simulink model "EuroNCAP_AEB_VRU_reversing_adult_stationary_cs"  (R2014b)
settings: Solver=ode5  SolverMode=SingleTasking  StartTime=0.0  StopTime=100  FixedStep=1/100  RelTol=1e-3
PreLoadFcn:
  | mbxruntime.callbacks.PreLoadFcn(bdroot);
  | check_NUTS_defined;
  | 
  | assignin('base',['model_closed_' bdroot],false);
  | 
  | addpath('../includes_PPS');
PostLoadFcn:
  | mbxruntime.callbacks.PostLoadFcn(bdroot);
InitFcn:
  | mbxruntime.callbacks.InitFcn(bdroot);
  | 
  | % Define simulink variables if they
  | % do not exist
  | if ~exist('HostVelocity', 'var')
  |   HostVelocity = 4;
  | end
  | 
  | if ~exist('Offset', 'var')
  |  Offset = 0;
  | end
StartFcn:
  | mbxruntime.callbacks.StartFcn(bdroot);
StopFcn:
  | mbxruntime.callbacks.StopFcn(bdroot);
model workspace: external: MAT-File .\EuroNCAP_AEB_VRU_reversing_adult_stationary_cs_hws.mat (data not in the file)
undefined symbols (not defined in the file or in its folder): mbxruntime, tabledata, warningInitialVelocity, x0
undefined symbols (not defined in the file): EuroNCAP_AEB_VRU_reversing_adult_stationary_cs_1d213d8ad9f41b81, EuroNCAP_AEB_VRU_reversing_adult_stationary_cs_23249e0323da09f5, EuroNCAP_AEB_VRU_reversing_adult_stationary_cs_24cc001f49944e92, EuroNCAP_AEB_VRU_reversing_adult_stationary_cs_285ecd3c3433122b, EuroNCAP_AEB_VRU_reversing_adult_stationary_cs_592b93520602ee78, EuroNCAP_AEB_VRU_reversing_adult_stationary_cs_7caeaf879e7765e9, EuroNCAP_AEB_VRU_reversing_adult_stationary_cs_93da770b460b611e, EuroNCAP_AEB_VRU_reversing_adult_stationary_cs_a0ea79e870de98f7, EuroNCAP_AEB_VRU_reversing_adult_stationary_cs_abfe9a01e22132d5, EuroNCAP_AEB_VRU_reversing_adult_stationary_cs_c7aa8805d7c8ab2f, EuroNCAP_AEB_VRU_reversing_adult_stationary_cs_c9a05fd8fd346e46, EuroNCAP_AEB_VRU_reversing_adult_stationary_cs_d44be614cd41bc1c, EuroNCAP_AEB_VRU_reversing_adult_stationary_cs_d8757d69723733e9, WheelL0, WheelL1, WheelR0, WheelR1
libraries: simulink x23, PreScanUsefulBlocks x19, simulink_extras x7, PreScanSimulinkLibrary x6
(part 1 of 5)
CloseFcn:
  | mbxruntime.callbacks.CloseFcn(bdroot);
  | evalin('base',['clear model_closed_' bdroot]);
settings Model: Creator=PRESCAN  LastModifiedBy=jenkins
settings DataIOCC: SignalLoggingSaveFormat=ModelDataLogs
settings OptimizationCC: InlineParams=on  ExpressionDepthLimit=2147483647  InitFltsAndDblsToZero=on
settings DebuggingCC: SaveWithParameterizedLinksMsg=none  UnderspecifiedInitializationDetection=Classic  MergeDetectMultiDrivingBlocksExec=none  SignalResolutionControl=TryResolveAllWithWarning  SolverPrmCheckMsg=none  MultiTaskDSMMsg=warning  MultiTaskCondExecSysMsg=none  FcnCallInpInsideContextMsg=UseLocalSettings  StateNameClashWarn=warning
settings ModelReferenceCC: UpdateModelReferenceTargets=IfOutOfDate
settings SFSimCC: SimParseCustomCode=off
settings SFSimCC: SimCustomHeaderCode=|
  | #include "prescan.h"
  | #include "prescan_platform.h"
settings RTWCC: IncludeERTFirstTime=on
settings GRTTargetCC: TargetFcnLib=ansi_tfl_tmw.mat  CombineOutputUpdateFcns=off  GRTInterface=on

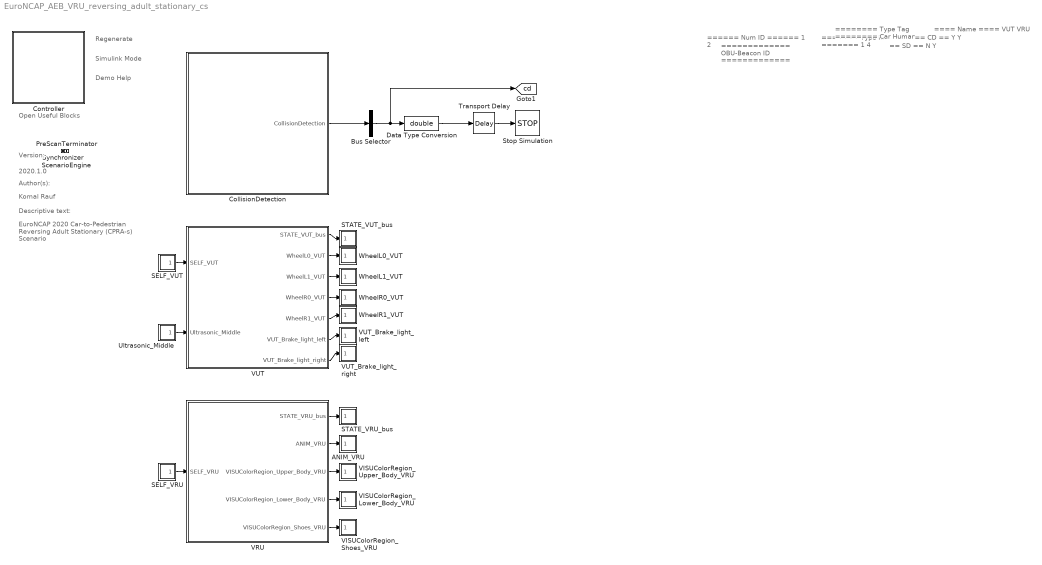
== system EuroNCAP_AEB_VRU_reversing_adult_stationary_cs ==
  note: Regenerate
  note: Simulink Mode
  note: Open Useful Blocks
  note: 2020.1.0
  note: Version:
  note: Author(s):
  note: Komal Rauf
  note: Descriptive text:
  note: EuroNCAP 2020 Car-to-Pedestrian
      | Reversing Adult Stationary
      | (CPRA-s) Scenario
  note: Demo Help
  note: ======
      | Num ID
      | ======
      | 1
      | 2
  note: =============
      | OBU-Beacon ID
      | =============
  note: =======
      | Type ID
      | =======
      | 1
      | 4
  note: ========
      | Type Tag
      | ========
      | Car
      | Human
  note: ==
      | SD
      | ==
      | N
      | Y
  note: ==
      | CD
      | ==
      | Y
      | Y
  note: ====
      | Name
      | ====
      | VUT
      | VRU
  ANIM_VRU : Subsystem  Tag=actuator/AnimationOutport  Priority=0  LoadFcn=load('PreScanAnimActuatorData.mat')  mask(PreScan Sink Block: State Animation){}
      mask help: The Human Animation port allows the human to walk, run or bend
      settings: OpenFcn=open_system([gcb '/Actuator'],'mask')
      mask Help: eval('openHelp(239)')
      mask Display: image(imread('HumanAnimated.jpg'))
  Bus Selector : BusSelector  OutputSignals=HEADER.valid
  CollisionDetection : Subsystem  Tag=sensor/CollisionDetection  Priority=30  LoadFcn=load('PrescanCollisionDetectionData.mat');load('PrescanCollisionDetectionMessage.mat')  mask(PreScan Source Block: CollisionDetection){}
      mask help: Collision Detection can be used to detect collisions between PreScan components. For Collision Detection the actual component shape is taken into account, so it is not a bounding box approach.
      settings: OpenFcn=open_system([gcb '/Sensor'],'mask')
      mask Help: eval('openHelp(811)')
      mask Display: image(imread('crash.jpg'))
  Controller : Subsystem  Description=8A3CD2955739A82C886C20AE3E253D78460D53180EE2C1B14CC08DF75A70BE77  Priority=-1  LoadFcn=load PreScanControllerData  mask(PreScan Simulation Controller){prescanversion='2020.1.0', ModelReferencing=off, TimeStep=1/100, ControlMode=0, PreScanExecutionMode=on, ControllerCount=0, ControllerIndex=0, ControllerOptions=''}
      mask prompts: prescanversion "PreScan Version"; ModelReferencing "Use Model Referencing"; TimeStep "Upload Period [s]"; ControlMode "Control Mode"; PreScanExecutionMode "Execution Mode"; ControllerCount "Controller Count"; ControllerIndex "Controller Index"; ControllerOptions "Controller Options"
      mask help:
      | Please do not remove this block from the compilation sheet,
      | as it connects the model to the PreScan environment.
      mask init:
      | model = bdroot(gcb);
      | ExperimentFile = mbxruntime.findExperimentFile(model,true); %relative path
      | 
      | [d1, d2, d3, prescandata] = prescan_Settings();
      | ModelDepo = fullfile(prescandata,'ModelDepo'); 
      | 
      | RTmode = mbxruntime.getRTMode(model);
      | 
      | SimulationMode = get_param(bdroot,'SimulationMode');
      | if strcmp(SimulationMode, 'rapid-accelerator')
      |     SimulationMode = 'external';
      | end
      | TargetName = get_param(bdroot,'SystemTargetFile');
      settings: ModelCloseFcn=assignin('base',['model_closed_' bdroot],true);
      mask Help: eval('openHelp(812)')
      mask Display: image(imread('prescanlogo.ico'))
  Data Type Conversion : DataTypeConversion  OutDataTypeStr=double
  PreScanTerminator : Subsystem  Tag=PreScanTerminator  Priority=999  LoadFcn=load PrescanTerminatorData  mask(PreScan Simulation Terminator){TimeStep=1/100}
      mask prompts: TimeStep "Upload Period [s]"
      mask help:
      | Please do not remove this block from the compilation sheet as it
      | connects the model to the PreScan environment.
      mask Help: eval('openHelp(812)')
      mask Display: image(imread('prescanlogo.ico'))
  SELF_VRU : Subsystem  Tag=sensor/SelfPort  Priority=30  LoadFcn=load('PreScanSelfSensorData.mat')  mask(PreScan Source Block: SELF){}
      mask help:
      | The SELF port shows (state) information of the actor itself. The outputs are position in the experiment's axis system and the GPS coordinates, and the object's absolute velocity and compass heading.
      |
      | For more information, please click Help.
      settings: OpenFcn=open_system([gcb '/Sensor'],'mask')
      mask Help: eval('openHelp(462)')
      mask Display: image(imread('GPS.png'))
  SELF_VUT : Subsystem  Tag=sensor/SelfPort  Priority=30  LoadFcn=load('PreScanSelfSensorData.mat')  mask(PreScan Source Block: SELF){}
      mask help:
      | The SELF port shows (state) information of the actor itself. The outputs are position in the experiment's axis system and the GPS coordinates, and the object's absolute velocity and compass heading.
      |
      | For more information, please click Help.
      settings: OpenFcn=open_system([gcb '/Sensor'],'mask')
      mask Help: eval('openHelp(462)')
      mask Display: image(imread('GPS.png'))
  STATE_VRU_bus : Subsystem  Tag=actuator/StatePort  Priority=0  LoadFcn=load('PreScanStateActuatorData.mat')  mask(PreScan Sink Block: State){}
      mask help:
      | The Actor State contains a vector signal of size (9x1), containing the following signals:
      |
      | -  Position    	(x,y,z)             	[m]
      | -  Velocity    	(vx,vy,vz)         	[m/s]
      | -  Angles       	(Roll, Pitch, Yaw)	[rad]
      |
      | The Actor state is defined in the global axis system.
      | The state is superponed on the Initial position defined in the GUI.
      |
      | For more information, please click Help.
      settings: OpenFcn=open_system([gcb '/Actuator'],'mask')
      mask Help: eval('openHelp(222)')
      mask Display: image(imread('State.png'))
  STATE_VUT_bus : Subsystem  Tag=actuator/StatePort  Priority=0  LoadFcn=load('PreScanStateActuatorData.mat')  mask(PreScan Sink Block: State){}
      mask help:
      | The Actor State contains a vector signal of size (9x1), containing the following signals:
      |
      | -  Position    	(x,y,z)             	[m]
      | -  Velocity    	(vx,vy,vz)         	[m/s]
      | -  Angles       	(Roll, Pitch, Yaw)	[rad]
      |
      | The Actor state is defined in the global axis system.
      | The state is superponed on the Initial position defined in the GUI.
      |
      | For more information, please click Help.
      settings: OpenFcn=open_system([gcb '/Actuator'],'mask')
      mask Help: eval('openHelp(222)')
      mask Display: image(imread('State.png'))
  ScenarioEngine : Subsystem  Tag=PreScanOpenScenarioBlock  Priority=10  LoadFcn=load PrescanSynchronizeData  mask(PreScan Simulation Core Block){TimeStep=1/100}
      mask prompts: TimeStep "Timestep [s]"
      mask help:
      | Please do not remove this block from the PreScan compilation sheet,
      | as it contains essential configuration parameters for a PreScan simulation.
      settings: DeleteFcn=PreScanBlockDeleteFcn;
      mask Display: image(imread('prescanlogo.ico'))
  Stop Simulation : Stop
  Synchronizer : Subsystem  Tag=PreScanSynchronizer  Priority=20  LoadFcn=load PrescanSynchronizeData  mask(PreScan Simulation Core Block){TimeStep=1/100}
      mask prompts: TimeStep "Timestep [s]"
      mask help:
      | Please do not remove this block from the PreScan compilation sheet,
      | as it contains essential configuration parameters for a PreScan simulation.
      settings: DeleteFcn=PreScanBlockDeleteFcn;
      mask Display: image(imread('prescanlogo.ico'))
  Transport Delay : TransportDelay  DelayTime=1/100
  Ultrasonic_Middle : Subsystem  Tag=sensor/UltraSonic  Priority=30  LoadFcn=load('PrescanScannerSensorData.mat');load('PrescanScannerSensorMessage.mat')  mask(PreScan Source Block: UltraSonic Sensor){}
      mask help:
      | The UltraSonic Sensor is a scanner device used to detect obstacles like cars, motor cycles, and pedestrians.
      |
      | For more information, please click Help.
      settings: OpenFcn=open_system([gcb '/Sensor'],'mask')
      mask Help: eval('openHelp(1465)')
      mask Display: image(imread('UltraSonic.png'))
  VISUColorRegion_Lower_Body_VRU : Subsystem  Tag=actuator/ColorRegion  Priority=0  LoadFcn=load('PrescanColorData')  mask(PreScan Sink Block: VisuTextureColor){}
      mask help:
      | The VisuTextureColor block provides a way to adapt the color of a vehicle.
      |
      | For more information, please click Help.
      settings: OpenFcn=open_system([gcb '/Actuator'],'mask')
      mask Help: eval('openHelp(230)')
      mask Display: image(imread('TextureColor.png'))
  VISUColorRegion_Shoes_VRU : Subsystem  Tag=actuator/ColorRegion  Priority=0  LoadFcn=load('PrescanColorData')  mask(PreScan Sink Block: VisuTextureColor){}
      mask help:
      | The VisuTextureColor block provides a way to adapt the color of a vehicle.
      |
      | For more information, please click Help.
      settings: OpenFcn=open_system([gcb '/Actuator'],'mask')
      mask Help: eval('openHelp(230)')
      mask Display: image(imread('TextureColor.png'))
  VISUColorRegion_Upper_Body_VRU : Subsystem  Tag=actuator/ColorRegion  Priority=0  LoadFcn=load('PrescanColorData')  mask(PreScan Sink Block: VisuTextureColor){}
      mask help:
      | The VisuTextureColor block provides a way to adapt the color of a vehicle.
      |
      | For more information, please click Help.
      settings: OpenFcn=open_system([gcb '/Actuator'],'mask')
      mask Help: eval('openHelp(230)')
      mask Display: image(imread('TextureColor.png'))
  VRU : Subsystem  Tag=WorldObjectSubSystem  InitFcn=UniqueId = '1024';
      mask init:
      | modelPath = GenericModelHelper.getGenericModelFilePath('ModelDepo','Humans\MaleRegular\Male_Regular.pgmb','f91824e3173f6a1007ae98b99b2fb1bd');imagePath = GenericModelHelper.getCompilationPicture(modelPath, 'MaleRegular.png');
      mask Display: image(imread(imagePath));color('white');text(0, 0, ' ID=2\n')
  VUT : Subsystem  Tag=WorldObjectSubSystem  InitFcn=UniqueId = '685';
      mask init:
      | modelPath = GenericModelHelper.getGenericModelFilePath('ModelDepo','Vehicles\Audi_A8\Audi_A8.pgmb','e33fe1ddcf3e8ae97caccbc8f2fa74ac');imagePath = GenericModelHelper.getCompilationPicture(modelPath, 'Audi_A8_HighPoly.png');
      mask Display: image(imread(imagePath));color('white');text(0, 0, ' ID=1\n')
  VUT_Brake_light_left : Subsystem  Tag=actuator/BrakeLightL  Priority=0  LoadFcn=load('PreScanVisuLightActuatorData');load('PrescanRPYData');load('PrescanXYZData');load('PreScanRGBData')  mask(PreScan Sink Block: VisuActiveLight){}
      mask help:
      | The VisuActiveLight block provides a way for detailed animation of Light Sources, such as the indicator, brake, fog and main lights of a vehicle, or a light post.
      |
      | For more information, please click Help.
      settings: OpenFcn=open_system([gcb '/Actuator'],'mask')
      mask Help: eval('openHelp(209)')
      mask Display: image(imread('HeadLight.png'))
  VUT_Brake_light_right : Subsystem  Tag=actuator/BrakeLightR  Priority=0  LoadFcn=load('PreScanVisuLightActuatorData');load('PrescanRPYData');load('PrescanXYZData');load('PreScanRGBData')  mask(PreScan Sink Block: VisuActiveLight){}
      mask help:
      | The VisuActiveLight block provides a way for detailed animation of Light Sources, such as the indicator, brake, fog and main lights of a vehicle, or a light post.
      |
      | For more information, please click Help.
      settings: OpenFcn=open_system([gcb '/Actuator'],'mask')
      mask Help: eval('openHelp(209)')
      mask Display: image(imread('HeadLight.png'))
  WheelL0_VUT : Subsystem  Tag=Actuator  Priority=0  LoadFcn=load('PrescanPoseData');load('PrescanXYZData');load('PreScanRPYData')
      mask help:
      | The VisuJoint block provides a way to adapt the location and orientation of a part of an object.
      |
      | For more information, please click Help.
      settings: OpenFcn=open_system([gcb '/Actuator'],'mask')
      mask Display: image(imread('Joint.png'))
  WheelL1_VUT : Subsystem  Tag=Actuator  Priority=0  LoadFcn=load('PrescanPoseData');load('PrescanXYZData');load('PreScanRPYData')
      mask help:
      | The VisuJoint block provides a way to adapt the location and orientation of a part of an object.
      |
      | For more information, please click Help.
      settings: OpenFcn=open_system([gcb '/Actuator'],'mask')
      mask Display: image(imread('Joint.png'))
  WheelR0_VUT : Subsystem  Tag=Actuator  Priority=0  LoadFcn=load('PrescanPoseData');load('PrescanXYZData');load('PreScanRPYData')
      mask help:
      | The VisuJoint block provides a way to adapt the location and orientation of a part of an object.
      |
      | For more information, please click Help.
      settings: OpenFcn=open_system([gcb '/Actuator'],'mask')
      mask Display: image(imread('Joint.png'))
  WheelR1_VUT : Subsystem  Tag=Actuator  Priority=0  LoadFcn=load('PrescanPoseData');load('PrescanXYZData');load('PreScanRPYData')
      mask help:
      | The VisuJoint block provides a way to adapt the location and orientation of a part of an object.
      |
      | For more information, please click Help.
      settings: OpenFcn=open_system([gcb '/Actuator'],'mask')
      mask Display: image(imread('Joint.png'))
  tag scope: cd=global
  wires:
  Bus Selector/1 -> Data Type Conversion/1, [cd]
  Data Type Conversion/1 -> Transport Delay/1
  Transport Delay/1 -> Stop Simulation/1
  CollisionDetection/1(CollisionDetection) -> Bus Selector/1
  VUT/1(STATE_VUT_bus) -> STATE_VUT_bus/1(STATE_VUT_bus)
  SELF_VUT/1(SELF_VUT) -> VUT/1(SELF_VUT)
  Ultrasonic_Middle/1(Ultrasonic_Middle) -> VUT/2(Ultrasonic_Middle)
  VUT/2(WheelL0_VUT) -> WheelL0_VUT/1(WheelL0_VUT)
  VUT/3(WheelL1_VUT) -> WheelL1_VUT/1(WheelL1_VUT)
  VUT/4(WheelR0_VUT) -> WheelR0_VUT/1(WheelR0_VUT)
  VUT/5(WheelR1_VUT) -> WheelR1_VUT/1(WheelR1_VUT)
  VUT/6(VUT_Brake_light_left) -> VUT_Brake_light_left/1(VUT_Brake_light_left)
  VUT/7(VUT_Brake_light_right) -> VUT_Brake_light_right/1(VUT_Brake_light_right)
  VRU/1(STATE_VRU_bus) -> STATE_VRU_bus/1(STATE_VRU_bus)
  VRU/2(ANIM_VRU) -> ANIM_VRU/1(ANIM_VRU)
  SELF_VRU/1(SELF_VRU) -> VRU/1(SELF_VRU)
  VRU/3(VISUColorRegion_Upper_Body_VRU) -> VISUColorRegion_Upper_Body_VRU/1(VISUColorRegion_Upper_Body_VRU)
  VRU/4(VISUColorRegion_Lower_Body_VRU) -> VISUColorRegion_Lower_Body_VRU/1(VISUColorRegion_Lower_Body_VRU)
  VRU/5(VISUColorRegion_Shoes_VRU) -> VISUColorRegion_Shoes_VRU/1(VISUColorRegion_Shoes_VRU)

== system EuroNCAP_AEB_VRU_reversing_adult_stationary_cs/ANIM_VRU ==
  ANIM_VRU : Inport  Tag=inport/AnimationOutport  OutDataTypeStr=Bus: PRESCAN_ANIMACTUATORDATA  PortDimensions=1  SampleTime=1/100  BusOutputAsStruct=on
  Actuator : S-Function  FunctionName=sfun_AnimActuator  Parameters=UniqueID, TimeStep  EnableBusSupport=off  mask(PreScan Sink Block: State Animation){UniqueID=1024, TimeStep=1/100}
      mask prompts: UniqueID "Auto-Assigned: Unique ID"; TimeStep "Auto-Assigned: Upload Period [s]"
      mask help: The Human Animation port allows the human to walk, run or bend
      mask Help: eval('openHelp(239)')
      mask Display: image(imread('HumanAnimated.jpg'))
  wires:
  ANIM_VRU/1 -> Actuator/1

== system EuroNCAP_AEB_VRU_reversing_adult_stationary_cs/CollisionDetection ==
  Sensor : S-Function  FunctionName=sfun_CollisionDetection  Parameters=detectableCollisions, timestep  EnableBusSupport=off  mask(PreScan Source Block: CollisionDetection){detectableCollisions=1, timestep=1/100}
      mask prompts: detectableCollisions "Max detectable collisions:"; timestep "MATLAB timestep:"
      mask help: Collision Detection can be used to detect collisions between PreScan components. For Collision Detection the actual component shape is taken into account, so it is not a bounding box approach.
      mask Help: eval('openHelp(811)')
      mask Display: image(imread('crash.jpg'))
  CollisionDetection : Outport  Tag=outport/CollisionDetection  OutDataTypeStr=Bus: PRESCAN_COLLISIONDETECTION_MESSAGE  PortDimensions=1  SampleTime=1/100
  wires:
  Sensor/1 -> CollisionDetection/1

== system EuroNCAP_AEB_VRU_reversing_adult_stationary_cs/Controller ==
  Terminator : Terminator
  sfun_Controller : S-Function  FunctionName=sfun_Controller  Parameters=SParameter1, SParameter2, SParameter3, SParameter4, SParameter5, SParameter6, SParameter7, SParameter8, SParameter9, SParameter10, SampleTime  EnableBusSupport=off  mask(Legacy Function){SFunctionSpec=void prescan_outputFcn(void** work1, PRESCAN_CONTROLLERDATA y1[1]), SParameter1=uint8([ExperimentFile 0]), SParameter2=uint8([ModelDepo 0]), SParameter3=uint8([ControllerOptions 0]), SParameter4=RTmode, SParameter5=PreScanExecutionMode, SParameter6=ControlMode, SParameter7=ControllerCount, SParameter8=ControllerIndex, SParameter9=uint8([SimulationMode 0]), SParameter10=uint8([TargetName 0]), SampleTime=TimeStep, ShowSpec=on}
      mask prompts: SParameter1 "P1:"; SParameter2 "P2:"; SParameter3 "P3:"; SParameter4 "P4:"; SParameter5 "P5:"; SParameter6 "P6:"; SParameter7 "P7:"; SParameter8 "P8:"; SParameter9 "P9:"; SParameter10 "P10:"; SampleTime "Sample time (-1 for inherited):"; ShowSpec "Display function specification"
      mask help:
      | This block allows you to call the legacy functions specified by the following Legacy Code Tool definition:
      | def.SFunctionName = 'sfun_Controller';
      | def.OutputFcnSpec = 'void prescan_outputFcn(void** work1, PRESCAN_CONTROLLERDATA y1[1])';
      | def.StartFcnSpec = 'void prescan_startFcn(void ** work1, uint8 p1[], uint8 p2[], uint8 p3[], double p4, double p5, double p6, double p7, double p8, uint8 p9[], uint8 p10[])';
      | def.TerminateFcnSpec = 'void prescan_terminateFcn(void** work1)';
      | def.HeaderFiles = {'prescan_controller_data.h', 'prescan_SFunLibrary.h', 'prescan_CreateLogHandler.h', 'prescan_CreateErrorHandler.h', 'prescan_modify.h', 'ModuleDLL.h'};
      | def.SourceFiles = {'prescan_MexLogHandler.c', 'prescan_SimStructErrorHandler.c', 'prescan_LogHandler.c', 'prescan_ErrorHandler.c', 'prescan_Modify.c'};
      | def.HostLibFiles = {'sensorinterfaced.lib'};
      | def.TargetLibFiles = {'sensorinterfaced.so'};
      | def.IncPaths = {'.', 'C:\projects\prescan\rt_vislibrary\vis\..\pimp\include\sensors\InterfaceRTW'};
      | def.SrcPaths = {'C:\projects\prescan\rt_vislibrary\vis\..\pimp\include\sensors\InterfaceRTW', 'C:\projects\prescan\rt_vislibrary\vis\..\pimp\include\sensors\InterfaceRTW\ccurrt'};
      | def.LibPaths = {'C:\\projects\\prescan\\vislibrary_build\lib'};
      | def.SampleTime = 'parameterized';
      mask Help: <p>This block was generated automatically by the Legacy Code Tool. For detailed help on this tool, call<a href="matlab:legacy_code('help')"> legacy_code('help')</a>.</p>
      mask Callback ShowSpec:
      | if strcmp(get_param(gcbh, 'ShowSpec'), 'on')
      |   set_param(gcbh, 'MaskDisplay', sprintf('fprintf(''%s'');', get_param(gcbh, 'SFunctionSpec')));
      | else
      |   set_param(gcbh, 'MaskDisplay', sprintf('fprintf(''%s'');', get_param(gcbh, 'FunctionName')));
      | end
      mask Display: fprintf('void prescan_outputFcn(void** work1, PRESCAN_CONTROLLERDATA y1[1])');
  wires:
  sfun_Controller/1 -> Terminator/1

== system EuroNCAP_AEB_VRU_reversing_adult_stationary_cs/PreScanTerminator ==
  Terminator : Terminator
  sfun_Terminator : S-Function  FunctionName=sfun_Terminator  Parameters=SampleTime  EnableBusSupport=off  mask(Legacy Function){SFunctionSpec=void prescan_terminator_outputFcn(void ** work1, PRESCAN_TERMINATORDATA y1[1]), SampleTime=TimeStep, ShowSpec=on}
      mask prompts: SampleTime "Sample time (-1 for inherited):"; ShowSpec "Display function specification"
      mask help:
      | This block allows you to call the legacy functions specified by the following Legacy Code Tool definition:
      | def.SFunctionName = 'sfun_Terminator';
      | def.OutputFcnSpec = 'void prescan_terminator_outputFcn(void ** work1, PRESCAN_TERMINATORDATA y1[1])';
      | def.StartFcnSpec = 'void prescan_terminator_startFcn(void ** work1)';
      | def.TerminateFcnSpec = 'void prescan_terminator_terminateFcn(void ** work1)';
      | def.HeaderFiles = {'prescan_terminator_data.h'};
      | def.HostLibFiles = {'sensorinterfaced.lib'};
      | def.IncPaths = {'src', 'C:\prescandev\vislibrary\vis\..\pimp\include\sensors\InterfaceRTW'};
      | def.SrcPaths = {'src'};
      | def.LibPaths = {'C:\\prescandev\\vislibrary_build\lib'};
      | def.SampleTime = 'parameterized';
      | def.Options.language = 'C';
      mask Help: <p>This block was generated automatically by the Legacy Code Tool. For detailed help on this tool, call<a href="matlab:legacy_code('help')"> legacy_code('help')</a>.</p>
      mask Callback ShowSpec:
      | if strcmp(get_param(gcbh, 'ShowSpec'), 'on')
      |   set_param(gcbh, 'MaskDisplay', sprintf('fprintf(''%s'');', get_param(gcbh, 'SFunctionSpec')));
      | else
      |   set_param(gcbh, 'MaskDisplay', sprintf('fprintf(''%s'');', get_param(gcbh, 'FunctionName')));
      | end
      mask Display: fprintf('void prescan_terminator_outputFcn(void ** work1, PRESCAN_TERMINATORDATA y1[1])');
  wires:
  sfun_Terminator/1 -> Terminator/1

== system EuroNCAP_AEB_VRU_reversing_adult_stationary_cs/SELF_VRU ==
  Sensor : S-Function  FunctionName=sfun_SelfSensor  Parameters=UniqueID, TimeStep  EnableBusSupport=off  mask(PreScan Source Block: SELF){UniqueID=1024, TimeStep=1/100}
      mask prompts: UniqueID "Auto-Assigned: Unique ID"; TimeStep "Auto-Assigned: Upload Period [s]"
      mask help:
      | The SELF port shows (state) information of the actor itself. The outputs are position in the experiment's axis system and the GPS coordinates, and the object's absolute velocity and compass heading.
      |
      | For more information, please click Help.
      mask Help: eval('openHelp(462)')
      mask Display: image(imread('GPS.png'))
  SELF_VRU : Outport  Tag=outport/SelfPort  OutDataTypeStr=Bus: PRESCAN_SELFSENSORDATA  PortDimensions=1  SampleTime=1/100
  wires:
  Sensor/1 -> SELF_VRU/1

== system EuroNCAP_AEB_VRU_reversing_adult_stationary_cs/SELF_VUT ==
  Sensor : S-Function  FunctionName=sfun_SelfSensor  Parameters=UniqueID, TimeStep  EnableBusSupport=off  mask(PreScan Source Block: SELF){UniqueID=685, TimeStep=1/100}
      mask prompts: UniqueID "Auto-Assigned: Unique ID"; TimeStep "Auto-Assigned: Upload Period [s]"
      mask help:
      | The SELF port shows (state) information of the actor itself. The outputs are position in the experiment's axis system and the GPS coordinates, and the object's absolute velocity and compass heading.
      |
      | For more information, please click Help.
      mask Help: eval('openHelp(462)')
      mask Display: image(imread('GPS.png'))
  SELF_VUT : Outport  Tag=outport/SelfPort  OutDataTypeStr=Bus: PRESCAN_SELFSENSORDATA  PortDimensions=1  SampleTime=1/100
  wires:
  Sensor/1 -> SELF_VUT/1

== system EuroNCAP_AEB_VRU_reversing_adult_stationary_cs/STATE_VRU_bus ==
  STATE_VRU_bus : Inport  Tag=inport/StatePort  OutDataTypeStr=Bus: PRESCAN_STATEACTUATORDATA  PortDimensions=1  SampleTime=1/100  BusOutputAsStruct=on
  Actuator : S-Function  FunctionName=sfun_StateActuator  Parameters=UniqueID, TimeStep  EnableBusSupport=off  mask(PreScan Sink Block: State){UniqueID=1024, TimeStep=1/100}
      mask prompts: UniqueID "Auto-Assigned: Unique ID"; TimeStep "Auto-Assigned: Upload Period [s]"
      mask help:
      | The Actor State contains a vector signal of size (9x1), containing the following signals:
      |
      | -  Position    	(x,y,z)             	[m]
      | -  Velocity    	(vx,vy,vz)         	[m/s]
      | -  Angles       	(Roll, Pitch, Yaw)	[rad]
      |
      | The Actor state is defined in the global axis system.
      | The state is superponed on the Initial position defined in the GUI.
      |
      | For more information, please click Help.
      mask Help: eval('openHelp(222)')
      mask Display: image(imread('State.png'))
  wires:
  STATE_VRU_bus/1 -> Actuator/1

== system EuroNCAP_AEB_VRU_reversing_adult_stationary_cs/STATE_VUT_bus ==
  STATE_VUT_bus : Inport  Tag=inport/StatePort  OutDataTypeStr=Bus: PRESCAN_STATEACTUATORDATA  PortDimensions=1  SampleTime=1/100  BusOutputAsStruct=on
  Actuator : S-Function  FunctionName=sfun_StateActuator  Parameters=UniqueID, TimeStep  EnableBusSupport=off  mask(PreScan Sink Block: State){UniqueID=685, TimeStep=1/100}
      mask prompts: UniqueID "Auto-Assigned: Unique ID"; TimeStep "Auto-Assigned: Upload Period [s]"
      mask help:
      | The Actor State contains a vector signal of size (9x1), containing the following signals:
      |
      | -  Position    	(x,y,z)             	[m]
      | -  Velocity    	(vx,vy,vz)         	[m/s]
      | -  Angles       	(Roll, Pitch, Yaw)	[rad]
      |
      | The Actor state is defined in the global axis system.
      | The state is superponed on the Initial position defined in the GUI.
      |
      | For more information, please click Help.
      mask Help: eval('openHelp(222)')
      mask Display: image(imread('State.png'))
  wires:
  STATE_VUT_bus/1 -> Actuator/1

== system EuroNCAP_AEB_VRU_reversing_adult_stationary_cs/ScenarioEngine ==
  Clock : Clock
  sfun_ScenarioEngine : S-Function  FunctionName=sfun_ScenarioEngine  Parameters=TimeStep  EnableBusSupport=off
  wires:
  Clock/1 -> sfun_ScenarioEngine/1

== system EuroNCAP_AEB_VRU_reversing_adult_stationary_cs/Synchronizer ==
  Bus Selector1 : BusSelector  OutputSignals=FederateStopped
  Stop Simulation : Stop
  sfun_Synchronizer : S-Function  FunctionName=sfun_Synchronizer  Parameters=SampleTime  EnableBusSupport=off  mask(Legacy Function){SFunctionSpec=void prescan_synchronizer_outputFcn(void ** work1, PRESCAN_SYNCHRONIZEDATA y1[1]), SampleTime=TimeStep, ShowSpec=on}
      mask prompts: SampleTime "Sample time (-1 for inherited):"; ShowSpec "Display function specification"
      mask help:
      | This block allows you to call the legacy functions specified by the following Legacy Code Tool definition:
      | def.SFunctionName = 'sfun_Synchronizer';
      | def.OutputFcnSpec = 'void prescan_synchronizer_outputFcn(void ** work1, PRESCAN_SYNCHRONIZEDATA y1[1])';
      | def.StartFcnSpec = 'void prescan_synchronizer_startFcn(void ** work1)';
      | def.TerminateFcnSpec = 'void prescan_synchronizer_terminateFcn(void ** work1)';
      | def.HeaderFiles = {'prescan_synchronizer_data.h'};
      | def.HostLibFiles = {'sensorinterfaced.lib'};
      | def.IncPaths = {'src', 'C:\prescandev\vislibrary\vis\..\pimp\include\sensors\InterfaceRTW'};
      | def.SrcPaths = {'src'};
      | def.LibPaths = {'C:\\prescandev\\vislibrary_build\lib'};
      | def.SampleTime = 'parameterized';
      | def.Options.language = 'C';
      mask Help: <p>This block was generated automatically by the Legacy Code Tool. For detailed help on this tool, call<a href="matlab:legacy_code('help')"> legacy_code('help')</a>.</p>
      mask Callback ShowSpec:
      | if strcmp(get_param(gcbh, 'ShowSpec'), 'on')
      |   set_param(gcbh, 'MaskDisplay', sprintf('fprintf(''%s'');', get_param(gcbh, 'SFunctionSpec')));
      | else
      |   set_param(gcbh, 'MaskDisplay', sprintf('fprintf(''%s'');', get_param(gcbh, 'FunctionName')));
      | end
      mask Display: fprintf('void prescan_synchronizer_outputFcn(void ** work1, PRESCAN_SYNCHRONIZEDATA y1[1])');
  wires:
  Bus Selector1/1 -> Stop Simulation/1  "<FederateStopped>"
  sfun_Synchronizer/1 -> Bus Selector1/1

== system EuroNCAP_AEB_VRU_reversing_adult_stationary_cs/Ultrasonic_Middle ==
  Sensor : S-Function  FunctionName=sfun_UltraSonic  Parameters=sensorID, detectableObjects, timestep  EnableBusSupport=off  mask(PreScan Source Block: UltraSonic Sensor){sensorID=690, detectableObjects=1, timestep=1/20}
      mask prompts: sensorID "Sensor ID"; detectableObjects "Max detectable objects:"; timestep "MATLAB timestep:"
      mask help:
      | The UltraSonic Sensor is a scanner device used to detect obstacles like cars, motor cycles, and pedestrians.
      |
      | For more information, please click Help.
      mask Help: eval('openHelp(1465)')
      mask Display: image(imread('UltraSonic.png'))
  Ultrasonic_Middle : Outport  Tag=outport/UltraSonic  OutDataTypeStr=Bus: PRESCAN_SCANNERSENSOR_MESSAGE  PortDimensions=1  SampleTime=1/20
  wires:
  Sensor/1 -> Ultrasonic_Middle/1

== system EuroNCAP_AEB_VRU_reversing_adult_stationary_cs/VISUColorRegion_Lower_Body_VRU ==
  VISUColorRegion_Lower_Body_VRU : Inport  Tag=inport/ColorRegion  OutDataTypeStr=Bus: PRESCAN_COLOR_DATA  PortDimensions=1  SampleTime=1/100  BusOutputAsStruct=on
  Actuator : S-Function  FunctionName=sfun_ColorActuator  Parameters=mbxruntime.parameters.convert(UniqueID), mbxruntime.parameters.convert(WorldModelSubPath),tabledata, TimeStep  EnableBusSupport=off  mask(PreScan Sink Block: VisuTextureColor){UniqueID=1024, WorldModelSubPath=/recolorRegion:name=Lower Body/targetColor, TimeStep=1/100}
      mask prompts: UniqueID "Parent Unique Identifier (auto-generated)"; WorldModelSubPath "WM SubPath(auto-generated)"; TimeStep "Simulink time step"
      mask help:
      | The VisuTextureColor block provides a way to adapt the color of a vehicle.
      |
      | For more information, please click Help.
      mask init:
      | [tabledata] = mbxruntime.parameters.table(UniqueID,WorldModelSubPath);
      mask Help: eval('openHelp(230)')
      mask Display: image(imread('TextureColor.png'))
  wires:
  VISUColorRegion_Lower_Body_VRU/1 -> Actuator/1

== system EuroNCAP_AEB_VRU_reversing_adult_stationary_cs/VISUColorRegion_Shoes_VRU ==
  VISUColorRegion_Shoes_VRU : Inport  Tag=inport/ColorRegion  OutDataTypeStr=Bus: PRESCAN_COLOR_DATA  PortDimensions=1  SampleTime=1/100  BusOutputAsStruct=on
  Actuator : S-Function  FunctionName=sfun_ColorActuator  Parameters=mbxruntime.parameters.convert(UniqueID), mbxruntime.parameters.convert(WorldModelSubPath),tabledata, TimeStep  EnableBusSupport=off  mask(PreScan Sink Block: VisuTextureColor){UniqueID=1024, WorldModelSubPath=/recolorRegion:name=Shoes/targetColor, TimeStep=1/100}
      mask prompts: UniqueID "Parent Unique Identifier (auto-generated)"; WorldModelSubPath "WM SubPath(auto-generated)"; TimeStep "Simulink time step"
      mask help:
      | The VisuTextureColor block provides a way to adapt the color of a vehicle.
      |
      | For more information, please click Help.
      mask init:
      | [tabledata] = mbxruntime.parameters.table(UniqueID,WorldModelSubPath);
      mask Help: eval('openHelp(230)')
      mask Display: image(imread('TextureColor.png'))
  wires:
  VISUColorRegion_Shoes_VRU/1 -> Actuator/1

== system EuroNCAP_AEB_VRU_reversing_adult_stationary_cs/VISUColorRegion_Upper_Body_VRU ==
  VISUColorRegion_Upper_Body_VRU : Inport  Tag=inport/ColorRegion  OutDataTypeStr=Bus: PRESCAN_COLOR_DATA  PortDimensions=1  SampleTime=1/100  BusOutputAsStruct=on
  Actuator : S-Function  FunctionName=sfun_ColorActuator  Parameters=mbxruntime.parameters.convert(UniqueID), mbxruntime.parameters.convert(WorldModelSubPath),tabledata, TimeStep  EnableBusSupport=off  mask(PreScan Sink Block: VisuTextureColor){UniqueID=1024, WorldModelSubPath=/recolorRegion:name=Upper Body/targetColor, TimeStep=1/100}
      mask prompts: UniqueID "Parent Unique Identifier (auto-generated)"; WorldModelSubPath "WM SubPath(auto-generated)"; TimeStep "Simulink time step"
      mask help:
      | The VisuTextureColor block provides a way to adapt the color of a vehicle.
      |
      | For more information, please click Help.
      mask init:
      | [tabledata] = mbxruntime.parameters.table(UniqueID,WorldModelSubPath);
      mask Help: eval('openHelp(230)')
      mask Display: image(imread('TextureColor.png'))
  wires:
  VISUColorRegion_Upper_Body_VRU/1 -> Actuator/1

== system EuroNCAP_AEB_VRU_reversing_adult_stationary_cs/VRU ==
  SELF_VRU : Inport  Tag=inport/SelfPort  OutDataTypeStr=Bus: PRESCAN_SELFSENSORDATA  PortDimensions=1  SampleTime=1/100  BusOutputAsStruct=on
  Animation : Subsystem  Tag=RunningHumanAnimation  mask(Prescan Conversion Block: Running Human Animation){MWS=1.95, WalkingScale=1.0, RunningScale=0.22, TimeStep=1/100}
      mask prompts: MWS "Maximum Walking Speed [m/s], above which the animation will switch to running mode."; WalkingScale "Walking mode scaling factor to sync the animation frames to the displacement."; RunningScale "Running mode scaling factor to sync the animation frames to the displacement."; TimeStep "Auto-Assigned: Upload Period [s]"
      mask help: The Running Human Animation block converts the State signal of a human into signals to properly control the animation.
      mask Help: eval('openHelp(239)');
      mask Display: image(imread('HumanAnimated.jpg'))
  ColorRegion_Lower_Body_color : Constant  Tag=VisuLightConst  Value=[0 0 255]
  ColorRegion_Shoes_color : Constant  Tag=VisuLightConst  Value=[0 0 0]
  ColorRegion_Upper_Body_color : Constant  Tag=VisuLightConst  Value=[165 42 42]
  Dynamics_Empty : Subsystem  Tag=Dynamics_Empty
      mask Help: eval('openHelp(202)')
      mask Display: port_label('output', 1, 'State');text(0,0,' Empty\n')
  SELF_Demux : Subsystem  Tag=demux/SelfPort  mask(PreScan Demux Block:){}
      mask help:
      | The SELF port shows (state) information of the actor itself. The outputs are position in the experiment's axis system and the GPS coordinates, and the object's absolute velocity and compass heading.
      |
      | For more information, please click Help.
      settings: DeleteFcn=PreScanBlockDeleteFcn;
      mask Help: eval('openHelp(462)')
      mask Display:
      | port_label('output',1,'x [m]')
      | port_label('output',2,'y [m]')
      | port_label('output',3,'z [m]','texmode','on')
      | port_label('output',4,'Rotx [deg]','texmode','on')
      | port_label('output',5,'Roty [deg]','texmode','on')
      | port_label('output',6,'Rotz [deg]','texmode','on')
      | port_label('output',7,'GPS lat [deg]','texmode','on')
      | port_label('output',8,'GPS long [deg]','texmode','on')
      | port_label('output',9,'GPS alt [m]','texmode','on')
      | port_label('output',10,'Velocity [m/s]')
      | port_label('output',11,'Heading [deg]')
      | port_label('output',12,'Yaw rate [deg/s]')
  STATE_VRU_rc : RateTransition  Tag=mux_rc/StatePort  OutPortSampleTimeOpt=Inherit
  Terminator_{1..12} (12 alike) : Terminator
  VISUColorRegion_Lower_Body_Mux : Subsystem  Tag=mux/MuxColorRegion  LoadFcn=load PrescanColorData  mask(PreScan User Interface: VisuTextureColor){}
      mask help:
      | The VisuTextureColor block provides a way to adapt the color of a vehicle.
      |
      | For more information, please click Help.
      settings: DeleteFcn=PreScanBlockDeleteFcn;
      mask Help: eval('openHelp(230)')
  VISUColorRegion_Shoes_Mux : Subsystem  Tag=mux/MuxColorRegion  LoadFcn=load PrescanColorData  mask(PreScan User Interface: VisuTextureColor){}
      mask help:
      | The VisuTextureColor block provides a way to adapt the color of a vehicle.
      |
      | For more information, please click Help.
      settings: DeleteFcn=PreScanBlockDeleteFcn;
      mask Help: eval('openHelp(230)')
  VISUColorRegion_Upper_Body_Mux : Subsystem  Tag=mux/MuxColorRegion  LoadFcn=load PrescanColorData  mask(PreScan User Interface: VisuTextureColor){}
      mask help:
      | The VisuTextureColor block provides a way to adapt the color of a vehicle.
      |
      | For more information, please click Help.
      settings: DeleteFcn=PreScanBlockDeleteFcn;
      mask Help: eval('openHelp(230)')
  STATE_VRU_bus : Outport  Tag=outport/StatePort  OutDataTypeStr=Bus: PRESCAN_STATEACTUATORDATA  PortDimensions=1  SampleTime=1/100
  ANIM_VRU : Outport  Tag=outport/AnimationOutport  Port=2  OutDataTypeStr=Bus: PRESCAN_ANIMACTUATORDATA  PortDimensions=1  SampleTime=1/100
  VISUColorRegion_Upper_Body_VRU : Outport  Tag=outport/ColorRegion  Port=3  OutDataTypeStr=Bus: PRESCAN_COLOR_DATA  PortDimensions=1  SampleTime=1/100
  VISUColorRegion_Lower_Body_VRU : Outport  Tag=outport/ColorRegion  Port=4  OutDataTypeStr=Bus: PRESCAN_COLOR_DATA  PortDimensions=1  SampleTime=1/100
  VISUColorRegion_Shoes_VRU : Outport  Tag=outport/ColorRegion  Port=5  OutDataTypeStr=Bus: PRESCAN_COLOR_DATA  PortDimensions=1  SampleTime=1/100
  wires:
  STATE_VRU_rc/1 -> STATE_VRU_bus/1
  Animation/1(Out1) -> ANIM_VRU/1
  SELF_VRU/1 -> SELF_Demux/1(SELF)
  VISUColorRegion_Upper_Body_Mux/1(ColorRegion) -> VISUColorRegion_Upper_Body_VRU/1
  ColorRegion_Upper_Body_color/1 -> VISUColorRegion_Upper_Body_Mux/1(RGB [-,-,-])
  VISUColorRegion_Lower_Body_Mux/1(ColorRegion) -> VISUColorRegion_Lower_Body_VRU/1
  ColorRegion_Lower_Body_color/1 -> VISUColorRegion_Lower_Body_Mux/1(RGB [-,-,-])
  VISUColorRegion_Shoes_Mux/1(ColorRegion) -> VISUColorRegion_Shoes_VRU/1
  ColorRegion_Shoes_color/1 -> VISUColorRegion_Shoes_Mux/1(RGB [-,-,-])
  Dynamics_Empty/1(State) -> STATE_VRU_rc/1, Animation/1(In1)
  SELF_Demux/1(x [m]) -> Terminator_1/1
  SELF_Demux/2(y [m]) -> Terminator_2/1
  SELF_Demux/3(z [m]) -> Terminator_3/1
  SELF_Demux/4(rotx [deg]) -> Terminator_4/1
  SELF_Demux/5(roty [deg]) -> Terminator_5/1
  SELF_Demux/6(rotz [deg]) -> Terminator_6/1
  SELF_Demux/7(GPS lat [deg]) -> Terminator_7/1
  SELF_Demux/8(GPS long [deg]) -> Terminator_8/1
  SELF_Demux/9(GPS alt [m]) -> Terminator_9/1
  SELF_Demux/10(velocity [m/s]) -> Terminator_10/1
  SELF_Demux/11(heading [deg]) -> Terminator_11/1
  SELF_Demux/12(yaw rate [deg/s]) -> Terminator_12/1
